simulink model "testMotors"  (Simulink 7.9)
settings: Solver=ode45  StartTime=0.0  StopTime=10.0  RelTol=1e-3
values from neighbouring files (symbols this model uses):
  m = canon(mot,'modal')    [HTenzoV1.m]    (also in HTenzoV2.m; HTenzoV3.m; HTenzoV4.m; HTenzoV5.m)
  m1 = canon(mot1,'modal')    [HTenzoV1.m]    (also in HTenzoV2.m; HTenzoV3.m; HTenzoV4.m; HTenzoV5.m)
undefined symbols (not defined in the file or in its folder): sigbuilder_block
settings Model: Creator=userk  LastModifiedBy=userk

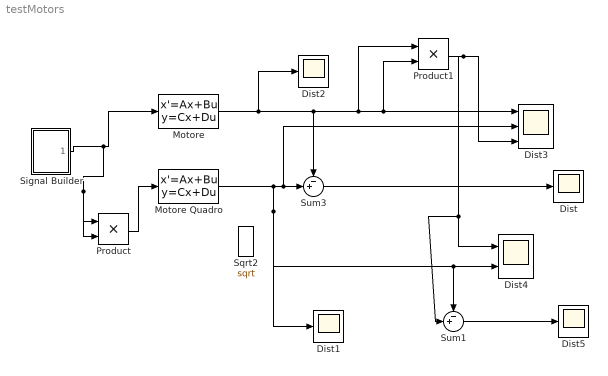
== system testMotors ==
  Dist{,1..2,5} (4 alike) : Scope
      Dist settings: TimeRange=15  YMin=-0.1  YMax=0.09
      Dist1 settings: TimeRange=15  YMin=-0.1  YMax=0.09
      Dist2 settings: TimeRange=15  YMin=-0.1  YMax=0.09  SaveName=ScopeData2
      Dist5 settings: TimeRange=15  YMin=-0.1  YMax=0.09  SaveName=ScopeData5
  Dist3 : Scope  NumInputPorts=3
      settings: TimeRange=15  YMin=-0.1~-5~-5  YMax=0.09~5~5  SaveName=ScopeData3
  Dist4 : Scope  NumInputPorts=2
      settings: TimeRange=15  YMin=-0.1~-5  YMax=0.09~5  SaveName=ScopeData4
  Motore : StateSpace  A=m.a  B=m.b  C=m.c  D=m.d
  Motore Quadro : StateSpace  A=m1.a  B=m1.b  C=m1.c  D=m1.d
  Product : Product  RndMeth=Zero
  Product1 : Product  RndMeth=Zero
  Signal Builder : Subsystem  Tag=STV Subsys  LoadFcn=sigbuilder_block('load');  StartFcn=sigbuilder_block('start');  StopFcn=sigbuilder_block('stop');  ClipboardFcn=sigbuilder_block('clipboard');  mask(Sigbuilder block){}
      mask help: Simulink:masks:SigbuilderBlock_MD
      mask init:
      | if ~strcmp(get_param(bdroot(gcbh),'SimulationStatus'),'stopped') tuvar = sigbuilder_block('maskInit'); end
      settings: CopyFcn=sigbuilder_block('copy');  DeleteFcn=sigbuilder_block('delete');  ModelCloseFcn=sigbuilder_block('modelClose');  PreSaveFcn=sigbuilder_block('preSave');  PauseFcn=sigbuilder_block('pause');  ContinueFcn=sigbuilder_block('continue');  NameChangeFcn=sigbuilder_block('namechange');  OpenFcn=sigbuilder_block('open',[341.6 120.8 550.4 400 ]);  CloseFcn=sigbuilder_block('close');
      mask Display: plot(0, 0, 100, 100,[2, 2, 32, 32, 2], [68, 8, 8, 68, 68],[32, 2], [38, 38], [32, 19, 2],[53, 60, 44], [32, 17, 17, 2],[16, 16, 31, 31]);txt = getActiveGroup(gcbh);text(2, 100, txt,'verticalAlignment', 'top');
  Sqrt2 : Sqrt  SaturateOnIntegerOverflow=on
  Sum1 : Sum  Inputs=-+|
  Sum3 : Sum  Inputs=-+|
  wires:
  Sum3/1 -> Dist/1
  Signal Builder/1(Signal 1) -> Motore/1, Product/1, Product/2
  Motore/1 -> Dist2/1, Sum3/1, Dist3/1, Product1/2, Product1/1
  Motore Quadro/1 -> Sum3/2, Dist3/2, Dist1/1, Dist4/2, Sum1/1
  Product/1 -> Motore Quadro/1
  Product1/1 -> Dist3/3, Dist4/1, Sum1/2
  Sum1/1 -> Dist5/1

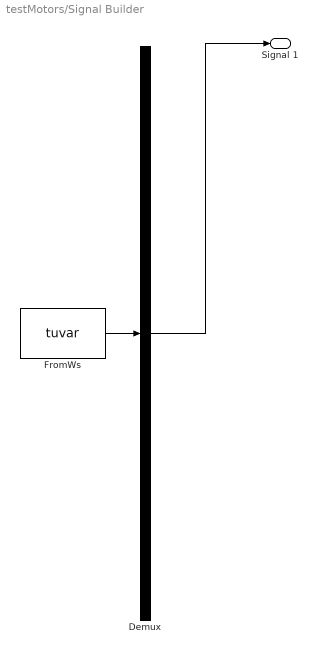
== system testMotors/Signal Builder ==
  Demux : Demux  Tag=STV Demux  Outputs=1
  FromWs : FromWorkspace  Tag=STV FromWs  VariableName=tuvar  SampleTime=0  SigBuilderData=DataTag0  VnvData=DataTag1
      SigBuilderData=|
      | common.afterFinalStr = 'Extrapolate'
      | common.sampleTime = 0
      | dataSet.timeRange = [0 10]
      | dataSet.name = 'Group 1'
      | sbobj.Groups.Name = 'Group 1'
      | sbobj.Groups.Signals.Name = 'Signal 1'
      | sbobj.Groups.Signals.XData = [0 4.06 4.06 6.82 6.82 10]
      | sbobj.Groups.Signals.YData = [190 1100 1910 1940 595 860]
  Signal 1 : Outport  Tag=STV Outport
  wires:
  Demux/1 -> Signal 1/1
  FromWs/1 -> Demux/1
